simulink model "ABS"  (R2020a)
settings: Solver=VariableStepAuto  StartTime=0.0  StopTime=10  RelTol=1e-3
values from neighbouring files (symbols this model uses):
  const = -g/4    (= -8.045)    [ABS_Datas.m]
  ctrl = 1    [ABS_Datas.m]
  I = 5    [ABS_Datas.m]
  Kf = 1    [ABS_Datas.m]    (also in Suspension_Datas.m = 28000)
  PBmax = 1500    [ABS_Datas.m]
  Rr = 1.25    [ABS_Datas.m]
  TB = 0.01    [ABS_Datas.m]
  Tt = u*m*g*Rr/4    (= 502.8125)    [ABS_Datas.m]
  v0 = 88    [ABS_Datas.m]
settings Model: Creator=Yogesh  LastModifiedBy=guru2

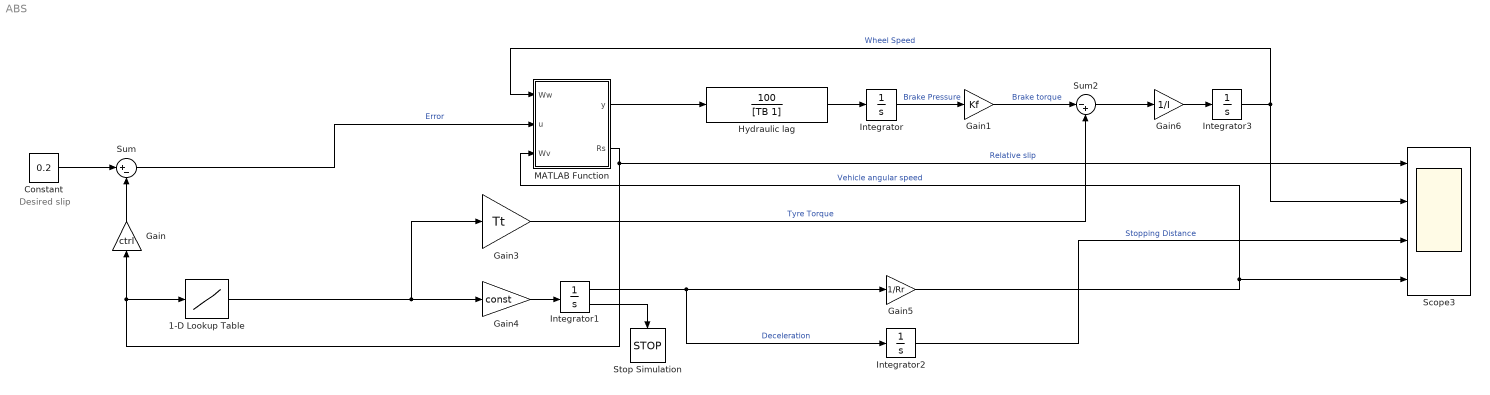
== system ABS ==
  note: Desired slip
  1-D Lookup Table : Lookup_n-D  NumberOfTableDimensions=1  BreakpointsForDimension1=[0,0.05,0.1,0.15,0.2,0.25,0.3,0.35,0.4,0.45,0.5,0.55,0.6,0.65,0.70,0.75,0.80,0.85,0.90,0.95,1]  Table=[0,.4,0.8,0.97,1,0.98,0.96,0.94,0.92,0.9,0.88,0.855,0.83,0.81,0.79,0.77,0.75,0.73,0.72,0.71,0.7]  InternalRulePriority=Speed  RndMeth=Simplest  InputSameDT=on
  Constant : Constant  Value=0.2
  Gain : Gain  Gain=ctrl
  Gain1 : Gain  Gain=Kf
  Gain3 : Gain  Gain=Tt
  Gain4 : Gain  Gain=const
  Gain5 : Gain  Gain=1/Rr
  Gain6 : Gain  Gain=1/I
  Hydraulic lag : TransferFcn  Numerator=[100]  Denominator=[TB 1]
  Integrator : Integrator  LimitOutput=on  UpperSaturationLimit=PBmax  LowerSaturationLimit=0
  Integrator1 : Integrator  InitialCondition=v0  LimitOutput=on  UpperSaturationLimit=1000  LowerSaturationLimit=0  ShowSaturationPort=on
  Integrator2 : Integrator
  Integrator3 : Integrator  InitialCondition=v0/Rr  LimitOutput=on  UpperSaturationLimit=1000  LowerSaturationLimit=0
  MATLAB Function : MATLAB Function  TreatAsAtomicUnit=on
  Scope3 : Scope  NumInputPorts=4
  Stop Simulation : Stop
  Sum : Sum  Inputs=|+-
  Sum2 : Sum  Inputs=|-+
  wires:
  Gain/1 -> Sum/2
  Constant/1 -> Sum/1
  Sum/1 -> MATLAB Function/2(u)  "Error"
  Hydraulic lag/1 -> Integrator/1
  Gain1/1 -> Sum2/1  "Brake torque"
  Integrator/1 -> Gain1/1  "Brake Pressure"
  1-D Lookup Table/1 -> Gain3/1, Gain4/1
  Gain3/1 -> Sum2/2  "Tyre Torque"
  Gain4/1 -> Integrator1/1
  Integrator1/2 -> Stop Simulation/1
  Integrator1/1 -> Integrator2/1, Gain5/1  "Deceleration"
  Gain5/1 -> MATLAB Function/3(Wv), Scope3/4  "Vehicle angular speed"
  Integrator2/1 -> Scope3/3  "Stopping Distance"
  Sum2/1 -> Gain6/1
  Gain6/1 -> Integrator3/1
  Integrator3/1 -> Scope3/2, MATLAB Function/1(Ww)  "Wheel Speed"
  MATLAB Function/2(Rs) -> Gain/1, 1-D Lookup Table/1, Scope3/1  "Relative slip"
  MATLAB Function/1(y) -> Hydraulic lag/1

== matlab function ABS/MATLAB Function ==
  data: Ww input; u input; y output; Wv input; Rs output
function [y,Rs] = fcn(Ww,u,Wv)
    Rs = 1-(Ww/Wv);
    if(u>0)
        y = 1;
    elseif (u<0)
        y = -1;
    else
        y = 0;
    end
end
